simulink model "system_sim"  (R2022b)
settings: Solver=FixedStepDiscrete  StartTime=0.0  StopTime=T_final  FixedStep=T_sample  RelTol=1e-3
values from neighbouring files (symbols this model uses):
  C_obsv_d = C_obsv    [run_model.m]
  D_obsv_d = D_obsv    [run_model.m]
  L_obsv = place(A_bar_d.',C_obsv_d.',P).'    [run_model.m]
  load_buses = [zeros(n_gen,1); ones(n_bus-n_gen,1)]    [run_model.m]
  n_bus = size(bus,1)    [run_model.m]
  n_gen = size(gen,1)    [run_model.m]
  n_states = 2*n_gen    [run_model.m]
  x0 = zeros(n_states,1)    [run_model.m]
undefined symbols (not defined in the file or in its folder): A_bar_d, B_bar_d, sigbuilder_block
libraries: simulink x1
settings Model: Creator=oanubi  LastModifiedBy=Abelb
settings SolverCC: AlgebraicLoopSolver=TrustRegion
settings DebuggingCC: UnconnectedInputMsg=warning  UnconnectedOutputMsg=warning  UnconnectedLineMsg=warning  SFMachineParentedDataDiag=warning
settings ModelReferenceCC: EnableRefExpFcnMdlSchedulingChecks=on
settings RTWCC: DLArmComputeVersion=19.05

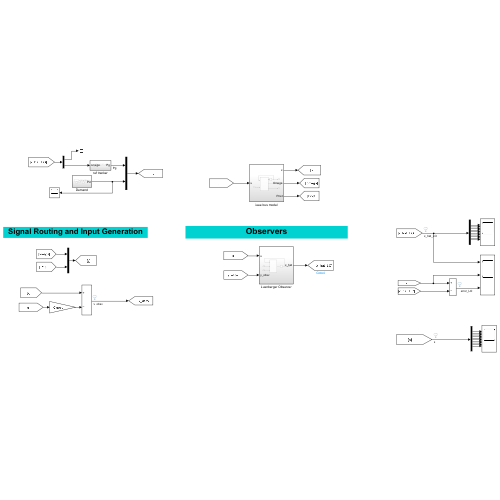
[thumbnail: Simulink's stored preview of the top-level diagram]
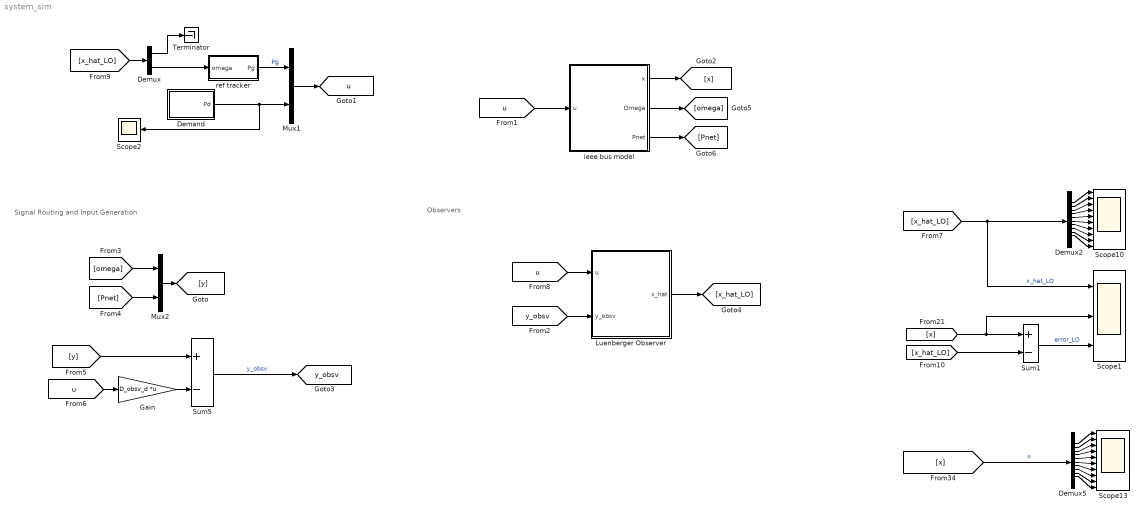
== system system_sim ==
  note: Signal Routing and Input Generation
  note: Observers
  Demand : Subsystem
  Demux : Demux  Outputs=2
  Demux2 : Demux  Outputs=n_states
  Demux5 : Demux  Outputs=n_states
  Gain : Gain  Gain=D_obsv_d  Multiplication=Matrix(K*u) (u vector)
  Luenberger Observer : Subsystem
  Mux1 : Mux  Inputs=2
  Mux2 : Mux  Inputs=2
  Scope1 : Scope  NumInputPorts=3
  Scope10 : Scope  NumInputPorts=10
  Scope13 : Scope  NumInputPorts=10
  Scope2 : Scope
  Sum1 : Sum  Inputs=+-
  Sum5 : Sum  Inputs=+-
  Terminator : Terminator
  ieee bus model : Subsystem
  ref tracker : Subsystem
  tag scope: u=global, y_obsv=global
  wires:
  Demux5/7 -> Scope13/7
  Gain/1 -> Sum5/2
  Demux2/7 -> Scope10/7
  Demand/1(Pd) -> Scope2/1, Mux1/2
  ieee bus model/2(Omega) -> [omega]
  Sum5/1 -> [y_obsv]  "y_obsv"
  Demux5/5 -> Scope13/5
  Demux2/10 -> Scope10/10
  Demux5/2 -> Scope13/2
  Demux/2 -> ref tracker/1(omega)
  [x] -> Sum1/1, Scope1/2
  Demux5/9 -> Scope13/9
  Demux2/3 -> Scope10/3
  Sum1/1 -> Scope1/3  "error_LO"
  Demux2/5 -> Scope10/5
  Demux2/1 -> Scope10/1
  Demux5/4 -> Scope13/4
  [y] -> Sum5/1
  Mux1/1 -> [u]
  [u] -> ieee bus model/1(u)
  Demux5/6 -> Scope13/6
  [u] -> Luenberger Observer/1(u)
  ieee bus model/1(x) -> [x]
  [y_obsv] -> Luenberger Observer/2(y_obsv)
  Demux5/3 -> Scope13/3
  Demux2/2 -> Scope10/2
  [x_hat_LO] -> Sum1/2
  Mux2/1 -> [y]
  Demux2/8 -> Scope10/8
  [x_hat_LO] -> Demux2/1, Scope1/1  "x_hat_LO"
  Demux5/8 -> Scope13/8
  Demux2/4 -> Scope10/4
  ref tracker/1(Pg) -> Mux1/1  "Pg"
  [omega] -> Mux2/1
  Demux2/6 -> Scope10/6
  ieee bus model/3(Pnet) -> [Pnet]
  Demux5/10 -> Scope13/10
  Demux5/1 -> Scope13/1
  Demux2/9 -> Scope10/9
  Luenberger Observer/1(x_hat) -> [x_hat_LO]
  [u] -> Gain/1
  [x] -> Demux5/1  "x"
  [Pnet] -> Mux2/2
  [x_hat_LO] -> Demux/1
  Demux/1 -> Terminator/1

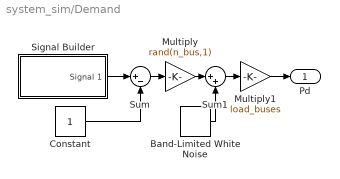
== system system_sim/Demand ==
  Band-Limited White Noise : simulink/Sources/Band-Limited White Noise  Cov=1e-8  Ts=0.1  seed=[23341]
  Constant : Constant
  Multiply : Gain  Gain=rand(n_bus,1)
  Multiply1 : Gain  Gain=load_buses
  Signal Builder : Subsystem  Tag=STV Subsys  LoadFcn=sigbuilder_block('load');  StartFcn=sigbuilder_block('start');  StopFcn=sigbuilder_block('stop');  ClipboardFcn=sigbuilder_block('clipboard');  mask(Sigbuilder block){tuvar=[0:10]}
      mask help: Simulink:masks:SigbuilderBlock_MD
      mask init:
      | if ~strcmp(get_param(bdroot(gcbh),'SimulationStatus'),'stopped') tuvar = sigbuilder_block('maskInit'); end
      settings: CopyFcn=sigbuilder_block('copy');  DeleteFcn=sigbuilder_block('delete');  ModelCloseFcn=sigbuilder_block('modelClose');  PreSaveFcn=sigbuilder_block('preSave');  PauseFcn=sigbuilder_block('pause');  ContinueFcn=sigbuilder_block('continue');  NameChangeFcn=sigbuilder_block('namechange');  OpenFcn=sigbuilder_block('open',[439.2 145.2 550.2 399.9 ]);  CloseFcn=sigbuilder_block('close');
      mask Display: plot(0, 0, 100, 100,[2, 2, 32, 32, 2], [68, 8, 8, 68, 68],[32, 2], [38, 38], [32, 19, 2],[53, 60, 44], [32, 17, 17, 2],[16, 16, 31, 31]);txt = getActiveGroup(gcbh);text(2, 100, txt,'verticalAlignment', 'top');
  Sum : Sum  Inputs=|+-
  Sum1 : Sum  Inputs=|++
  Pd : Outport
  wires:
  Sum/1 -> Multiply/1
  Signal Builder/1(Signal 1) -> Sum/1
  Constant/1 -> Sum/2
  Multiply/1 -> Sum1/1
  Band-Limited White Noise/1 -> Sum1/2
  Sum1/1 -> Multiply1/1
  Multiply1/1 -> Pd/1

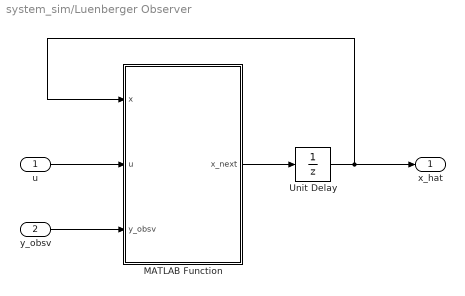
== system system_sim/Luenberger Observer ==
  u : Inport
  y_obsv : Inport  Port=2
  MATLAB Function : MATLAB Function  TreatAsAtomicUnit=on
  Unit Delay : UnitDelay  InitialCondition=zeros(n_states,1)  SampleTime=-1  HasFrameUpgradeWarning=on
  x_hat : Outport
  wires:
  MATLAB Function/1(x_next) -> Unit Delay/1
  Unit Delay/1 -> x_hat/1, MATLAB Function/1(x)
  u/1 -> MATLAB Function/2(u)
  y_obsv/1 -> MATLAB Function/3(y_obsv)

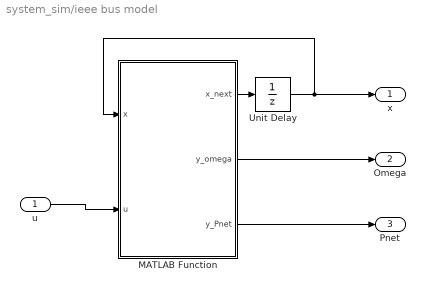
== system system_sim/ieee bus model ==
  u : Inport
  MATLAB Function : MATLAB Function  TreatAsAtomicUnit=on
  Unit Delay : UnitDelay  InitialCondition=x0  SampleTime=-1  HasFrameUpgradeWarning=on
  x : Outport
  Omega : Outport  Port=2
  Pnet : Outport  Port=3
  wires:
  MATLAB Function/1(x_next) -> Unit Delay/1
  Unit Delay/1 -> x/1, MATLAB Function/1(x)
  u/1 -> MATLAB Function/2(u)
  MATLAB Function/2(y_omega) -> Omega/1
  MATLAB Function/3(y_Pnet) -> Pnet/1

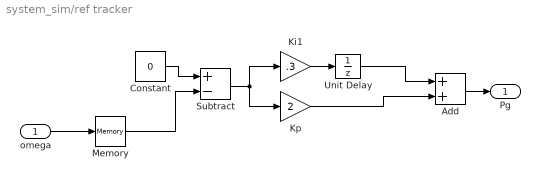
== system system_sim/ref tracker ==
  omega : Inport
  Add : Sum
  Constant : Constant  Value=0
  Ki1 : Gain  Gain=.3
  Kp : Gain  Gain=2
  Memory : Memory  InitialCondition=zeros(n_gen,1)
  Subtract : Sum  Inputs=+-
  Unit Delay : UnitDelay  InitialCondition=zeros(n_gen,1)  SampleTime=-1  HasFrameUpgradeWarning=on
  Pg : Outport
  wires:
  Kp/1 -> Add/2
  Unit Delay/1 -> Add/1
  Add/1 -> Pg/1
  Constant/1 -> Subtract/1
  Subtract/1 -> Ki1/1, Kp/1
  Ki1/1 -> Unit Delay/1
  Memory/1 -> Subtract/2
  omega/1 -> Memory/1

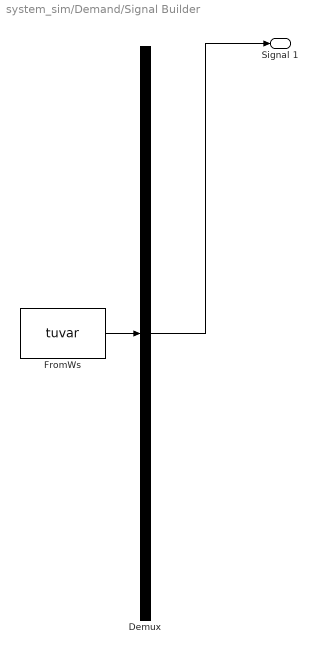
== system system_sim/Demand/Signal Builder ==
  Demux : Demux  Tag=STV Demux  Outputs=1
      settings: DisplayOption=none
  FromWs : FromWorkspace  Tag=STV FromWs  VariableName=tuvar
      SigBuilderData=|
      | common.afterFinalStr = 'Extrapolate'
      | common.sampleTime = 0
      | dataSet.timeRange = [0 10]
      | dataSet.name = 'Group 1'
      | sbobj.Groups.Name = 'Group 1'
      | sbobj.Groups.Signals.Name = 'Signal 1'
      | sbobj.Groups.Signals.XData = [0 0.46 1.5 2.5 4 5 6 7 10]
      | sbobj.Groups.Signals.YData = [1 1.106 1.2 1.2 0.8 0.8 1 1 1]
  Signal 1 : Outport  Tag=STV Outport
  wires:
  Demux/1 -> Signal 1/1
  FromWs/1 -> Demux/1

== matlab function system_sim/Luenberger Observer/MATLAB Function ==
  data: x input; x_next output; u input; y_obsv input; L_obsv parameter; A_bar_d parameter; C_obsv_d parameter; B_bar_d parameter
function x_next  = fcn(x,u,y_obsv,L_obsv,A_bar_d,C_obsv_d,B_bar_d)
% Discrete state-space model for system

x_next = A_bar_d*x + B_bar_d*u + L_obsv*(y_obsv - C_obsv_d*x);

== matlab function system_sim/ieee bus model/MATLAB Function ==
  data: x input; x_next output; u input; y_omega output; A_bar_d parameter; C_obsv_d parameter; B_bar_d parameter; D_obsv_d parameter; n_gen parameter; n_bus parameter; y_Pnet output
function [x_next,y_omega,y_Pnet] = fcn(x,u,A_bar_d,C_obsv_d,B_bar_d,D_obsv_d,n_gen, n_bus)
% Discrete state-space model for system

x_next = A_bar_d*x + B_bar_d*u;

y = C_obsv_d*x + D_obsv_d*u;

y_omega = y(1:n_gen);
y_Pnet = y(n_gen+1:n_bus+n_gen);
